simulink model "Q1F_LinearX"  (R2015b)
settings: Solver=VariableStepAuto  StartTime=0.0  StopTime=100  RelTol=1e-3
values from neighbouring files (symbols this model uses):
  A = [ 0, 1,                  0, 0,                      0, 0 ... (first row only)    [Q1E.m]    (also in Q1F_Init_Models_Overall.m = [ 0, 1,               0,     0,              0, 0; Q1F_Init_Models_x.m = [ 0, 1,               0,     0,              0, 0; Q1F_Init_Models_xQ1Q2.m = [ 0, 1,               0,     0,              0, 0; Q1F_Init_Models_xQ2.m = [ 0, 1,               0,     0,              0, 0)
  Ax_obs = [A-Lx*Cx]    [Q1F_Init_Models_Overall.m]    (also in Q1F_Init_Models_x.m)
  B = [  0 ... (first row only)    [Q1E.m]    (also in Q1F_Init_Models_Overall.m = [ 0; Q1F_Init_Models_x.m = [ 0; Q1F_Init_Models_xQ1Q2.m = [ 0; Q1F_Init_Models_xQ2.m = [ 0)
  Bx_obs = [B Lx]    [Q1F_Init_Models_Overall.m]    (also in Q1F_Init_Models_x.m)
  C_all = eye(6)    [Q1F_Init_Models_Overall.m]    (also in Q1F_Init_Models_x.m; Q1F_Init_Models_xQ1Q2.m; Q1F_Init_Models_xQ2.m; Q1G_Init_Model.m)
  Cx = [1 0 0 0 0 0]    [Q1F_Init_Models_Overall.m]    (also in Q1F_Init_Models_x.m; Q1G_Init_Model.m)
  D = zeros(6,1)    [Q1E.m]    (also in Q1F_Init_Models_Overall.m; Q1F_Init_Models_x.m; Q1F_Init_Models_xQ1Q2.m; Q1F_Init_Models_xQ2.m)
  Dx_obs = [0 0; 0 0; 0 0; 0 0; 0 0; 0 0]    [Q1F_Init_Models_Overall.m]    (also in Q1F_Init_Models_x.m)
  X_0_l = [0 0 X_0(3)*pi/180 X_0(4)*pi/180 X_0(5)*pi/180 X_0(6)*pi/180]'    [Q1E.m]    (also in Q1F_Init_Models_Overall.m = [X_0(1) X_0(2) X_0(3)*pi/180 X_0(4)*pi/180 X_0(5)*pi/180 X_0; Q1F_Init_Models_x.m = [X_0(1) X_0(2) X_0(3)*pi/180 X_0(4)*pi/180 X_0(5)*pi/180 X_0; Q1F_Init_Models_xQ1Q2.m = [X_0(1) X_0(2) X_0(3)*pi/180 X_0(4)*pi/180 X_0(5)*pi/180 X_0; Q1F_Init_Models_xQ2.m = [X_0(1) X_0(2) X_0(3)*pi/180 X_0(4)*pi/180 X_0(5)*pi/180 X_0)
  X_0_x_obs = [0 0 0 0 0 0]    [Q1F_Init_Models_Overall.m]    (also in Q1F_Init_Models_x.m)
undefined symbols (not defined in the file or in its folder): K
settings Model: Creator=Chirag  LastModifiedBy=ANKUR

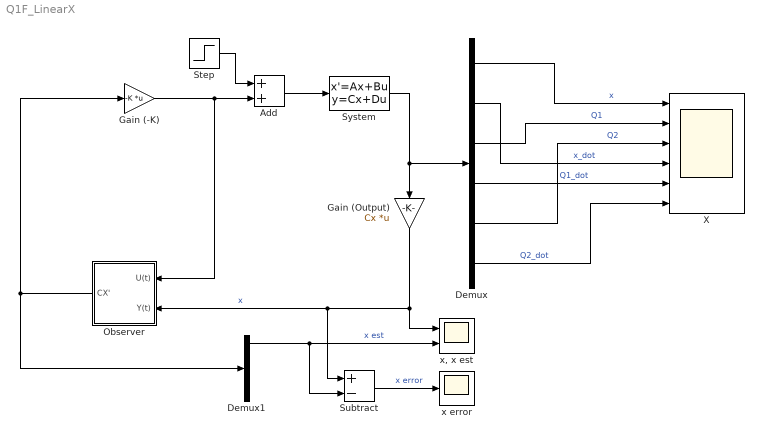
== system Q1F_LinearX ==
  Add : Sum
  Demux : Demux  Outputs=6
  Demux1 : Demux  Outputs=6
  Gain (-K) : Gain  Gain=-K  Multiplication=Matrix(K*u) (u vector)
  Gain (Output) : Gain  Gain=Cx  Multiplication=Matrix(K*u)
  Observer : Subsystem
  Step : Step  Time=0  SampleTime=0
  Subtract : Sum  Inputs=+-
  System : StateSpace  A=A  B=B  C=C_all  D=D  X0=X_0_l
  X : Scope  NumInputPorts=6
  x error : Scope
  "x, x est" : Scope  NumInputPorts=2
  wires:
  System/1 -> Gain (Output)/1, Demux/1
  Observer/1(CX') -> Gain (-K)/1, Demux1/1
  Gain (Output)/1 -> "x, x est"/1, Subtract/1, Observer/2(Y(t))  "x"
  Gain (-K)/1 -> Observer/1(U(t)), Add/2
  Add/1 -> System/1
  Step/1 -> Add/1
  Demux1/1 -> Subtract/2, "x, x est"/2  "x est"
  Demux/1 -> X/1  "x"
  Demux/3 -> X/2  "Q1"
  Demux/5 -> X/3  "Q2"
  Demux/2 -> X/4  "x_dot"
  Demux/4 -> X/5  "Q1_dot"
  Demux/6 -> X/6  "Q2_dot"
  Subtract/1 -> x error/1  "x error"

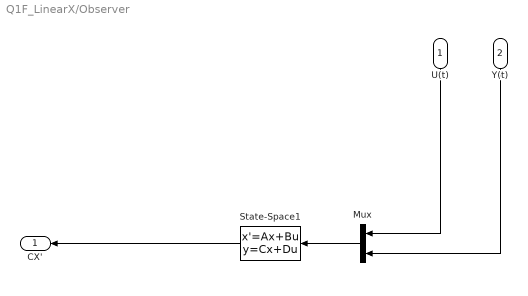
== system Q1F_LinearX/Observer ==
  U(t) : Inport
  Y(t) : Inport  Port=2
  Mux : Mux  Inputs=2
  State-Space1 : StateSpace  A=Ax_obs  B=Bx_obs  C=C_all  D=Dx_obs  X0=X_0_x_obs
  CX' : Outport
  wires:
  State-Space1/1 -> CX'/1
  Y(t)/1 -> Mux/2
  Mux/1 -> State-Space1/1
  U(t)/1 -> Mux/1
